simulink model "JOLT"  (R2023a)
settings: Solver=FixedStepAuto  StartTime=0.0  StopTime=2000  RelTol=1e-3
model workspace (MAT data in the model file):
  SampleTime = 0.001
  T_npxls = 4
  T_pupil = 100
  T_whisk = 20
  maxFrames = 60000
  tStop = 1800
  toneDuration = 1.5
undefined symbols (not defined in the file or in its folder): Ended, Single
libraries: speedgoatlib_IO191 x4, slrealtimeiplib x3
settings Model: Creator=electro  LastModifiedBy=electro
settings SolverCC: ConcurrentTasks=on  PositivePriorityOrder=on  AutoInsertRateTranBlk=on
settings DataIOCC: SaveFormat=Array
settings OptimizationCC: BlockReduction=off  OptimizeBlockIOStorage=off  EnhancedBackFolding=on  PassReuseOutputArgsThreshold=0  OptimizeBlockOrder=speed  DifferentSizesBufferReuse=on
settings DebuggingCC: TasksWithSamePriorityMsg=none  ParameterTunabilityLossMsg=error  SFUnexpectedBacktrackingDiag=warning  SFNoUnconditionalDefaultTransitionDiag=warning  UnderSpecifiedDimensionMsg=warning
settings HardwareCC: ProdBitPerLong=64  ProdLongLongMode=on  ProdHWDeviceType=Intel->x86-64 (Linux 64)
settings SFSimCC: SimUserIncludeDirs="\"/usr/local/MATLAB/R2023a/toolbox/slrealtime/target/kernel/dist/include/verify\""
settings RTWCC: Description=Simulink Real-Time  SystemTargetFile=slrealtime.tlc  TemplateMakefile=slrealtime_default_tmf  GenerateReport=on  RTWVerbose=off  CustomInclude=/usr/local/MATLAB/R2023a/toolbox/slrealtime/target/kernel/dist/include,  Toolchain=Simulink Real-Time Toolchain  BuildConfiguration=Faster Runs  CodeExecutionProfiling=on  TargetLang=C++
settings CodeAppCC: ForceParamTrailComments=on  OperatorAnnotations=on  EnableCustomComments=on

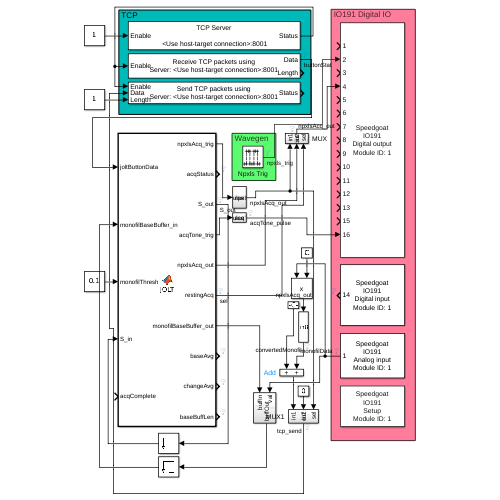
[thumbnail: Simulink's stored preview of the top-level diagram]
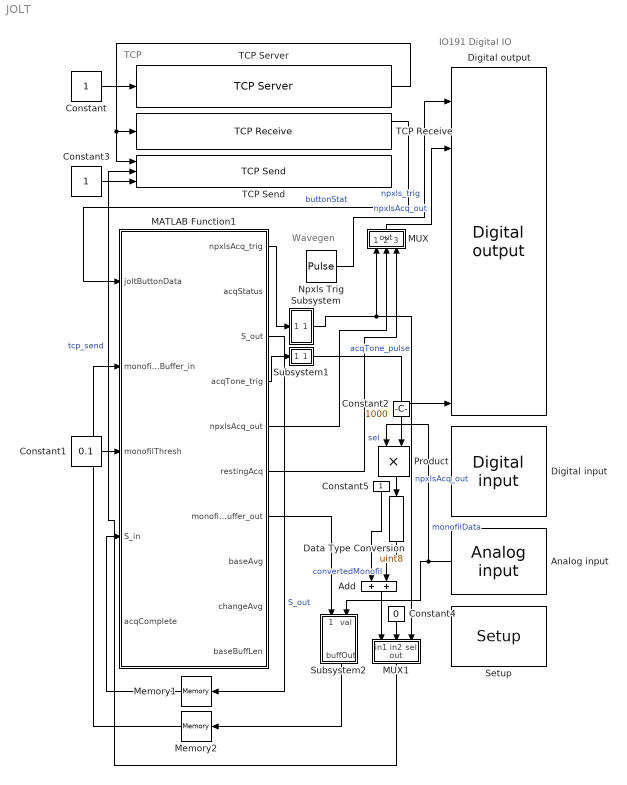
== system JOLT ==
  note: Wavegen
  note: TCP
  note: IO191 Digital IO
  Add : Sum
  "Analog input " : speedgoatlib_IO191/Analog input   parModuleId=1  parSampleTime=SampleTime  parPciSlot=-1  parAdcChannels=1  parAdcMode=2  parAdcRanges=4  parAdcRate=100000  parAdcInitValues=[0 0]  parAdcResets=[1 1]
      settings: SourceProductName=Simulink Real-Time: Speedgoat I/O Blockset
  Constant : Constant
  Constant1 : Constant  Value=0.1
  Constant2 : Constant  Value=1000
  Constant3 : Constant
  Constant4 : Constant  Value=0
  Constant5 : Constant
  Data Type Conversion : DataTypeConversion  OutMin=1  OutMax=255  OutDataTypeStr=uint8  RndMeth=Ceiling  SaturateOnIntegerOverflow=off
  "Digital input " : speedgoatlib_IO191/Digital input   parModuleId=1  parSampleTime=SampleTime  parPciSlot=-1  parDiChannels=14
      settings: SourceProductName=Simulink Real-Time: Speedgoat I/O Blockset
  "Digital output " : speedgoatlib_IO191/Digital output   parModuleId=1  parSampleTime=SampleTime  parPciSlot=-1  parDoChannels=[1 2 3 4 5 6 7 8 9 10 11 12 13 15 16]  parDoInitValues=[1 0 0 0 0 0 0 0 0 0 0 0 0 0 0]  parDoResets=[1 1 1 1 1 1 1 1 1 1 1 1 1 1 1]
      settings: SourceProductName=Simulink Real-Time: Speedgoat I/O Blockset
  MATLAB Function1 : MATLAB Function  TreatAsAtomicUnit=on
  MUX : Subsystem
  MUX1 : Subsystem
  Memory1 : Memory  InheritSampleTime=on
  Memory2 : Memory  InheritSampleTime=on
  Npxls Trig : DiscretePulseGenerator  Amplitude=2.5  Period=T_npxls  PulseWidth=T_npxls/2  SampleTime=SampleTime
  Product : Product
  "Setup " : speedgoatlib_IO191/Setup   parModuleId=1  parPciSlot=-1  parTriggerSignal=TTL  parAdcChannels=1  parAdcRanges=4  parAdcChannel1=on  parAdcChannel2=off  parAdcChannel3=off  parAdcChannel4=off  parAdcChannel5=off  parAdcChannel6=off  parAdcChannel7=off  parAdcChannel8=off  parAdcMode=Single-Ended  parAdcRate=100000  parAdcRange11=+-5.12 V  parAdcRange21=+-24.576 V  parAdcRange12=+-10.24 V  parAdcRange22=+-24.576 V  parAdcRange13=+-10.24 V  parAdcRange23=+-24.576 V  parAdcRange14=+-10.24 V  parAdcRange24=+-24.576 V  parAdcRange15=+-10.24 V  parAdcRange25=+-24.576 V  parAdcRange16=+-10.24 V  parAdcRange26=+-24.576 V  parAdcRange17=+-10.24 V  parAdcRange27=+-24.576 V  parAdcRange18=+-10.24 V  parAdcRange28=+-24.576 V  parDacChannels=[1 2]  parDacChannel1=on  parDacChannel2=on  parDacChannel3=off  parDacChannel4=off  parDacMode=Single-Ended  parDacRanges=[4 4]  parDacInitValues=[0 0]  parDacResets=[1 1]  parDacRange1=+-10 V  parDacInitValue1=0  parDacReset1=on  parDacRange2=+-10 V  parDacInitValue2=0  parDacReset2=on  parDacRange3=+-10 V  parDacInitValue3=0  parDacReset3=on  parDacRange4=+-10 V  parDacInitValue4=0  parDacReset4=on  parDiChannels=14  parDoChannels=[1 2 3 4 5 6 7 8 9 10 11 12 13 15 16]  parDioFirstControl=[1 2 3 4 5 6 8 9]  parDioSecondControl=0  parDioChannel1=Out  parExtra1=I  parExtra2=I  parExtra3=I  parDioChannel2=Out  parDioChannel3=Out  parDioChannel4=Out  parDioChannel5=Out  parDioChannel6=Out  parDioChannel7=In  parDioChannel8=Out  parDioChannel9=Out  parDoInitValues=[0 0 0 0]  parDoResets=[1 1 1 1]  parDoInitValue1=1  parDoReset1=on  parDoInitValue2=0  parDoReset2=on  parDoInitValue3=0  parDoReset3=on  parDoInitValue4=0  parDoReset4=on  parDoInitValue5=0  parDoReset5=on  parDoInitValue6=0  parDoReset6=on  parDoInitValue7=0  parDoReset7=on  parDoInitValue8=0  parDoReset8=on  parDoInitValue9=0  parDoReset9=on  parDoInitValue10=0  parDoReset10=on  parDoInitValue11=0  parDoReset11=on  parDoInitValue12=0  parDoReset12=on  parDoInitValue13=0  parDoReset13=on  parDoInitValue14=0  parDoReset14=on  parDoInitValue15=0  parDoReset15=on  parDoInitValue16=0  parDoReset16=on
      settings: SourceProductName=Simulink Real-Time: Speedgoat I/O Blockset
  Subsystem : Subsystem
  Subsystem1 : Subsystem
  Subsystem2 : Subsystem
  TCP Receive : slrealtimeiplib/TCP Receive  socketAddPortVal=Server: <Use host-target connection>:8001  rcvWidth=1  sampleTime=SampleTime
  TCP Send : slrealtimeiplib/TCP Send  socketAddPortVal=Server: <Use host-target connection>:8001  sampleTime=SampleTime
  TCP Server : slrealtimeiplib/TCP Server  Priority=-1  useHostTargetConn=on  serverAddress=10.10.10.15  serverPort=8001
  wires:
  TCP Receive/1 -> MATLAB Function1/1(joltButtonData)  "buttonStat"
  TCP Server/1 -> TCP Send/1, TCP Receive/1
  Constant/1 -> TCP Server/1
  Npxls Trig/1 -> "Digital output "/2  "npxls_trig"
  "Analog input "/1 -> Subsystem2/2(val), Product/1  "monofilData"
  MATLAB Function1/3(S_out) -> Memory1/1  "S_out"
  Memory1/1 -> MATLAB Function1/4(S_in)
  MATLAB Function1/4(acqTone_trig) -> Subsystem1/1(acqTone_trig)
  Subsystem1/1(sigPulse) -> "Digital output "/15  "acqTone_pulse"
  Constant1/1 -> MATLAB Function1/3(monofilThresh)
  MUX/1(out) -> "Digital output "/4  "npxlsAcq_out"
  Subsystem/1(sigPulse) -> MUX1/3(sel), MUX/1(in1)  "npxlsAcq_out"
  MATLAB Function1/5(npxlsAcq_out) -> MUX/2(in2)
  MATLAB Function1/6(restingAcq) -> MUX/3(sel)  "sel"
  MATLAB Function1/1(npxlsAcq_trig) -> Subsystem/1(npxlsAcq_trig)
  MATLAB Function1/7(monofilBaseBuffer_out) -> Subsystem2/1(buffIn)
  Subsystem2/1(buffOut) -> Memory2/1
  Memory2/1 -> MATLAB Function1/2(monofilBaseBuffer_in)
  Constant2/1 -> Product/2
  Constant3/1 -> TCP Send/3
  Constant4/1 -> MUX1/2(in2)
  MUX1/1(out) -> TCP Send/2  "tcp_send"
  Constant5/1 -> Add/1
  Product/1 -> Data Type Conversion/1
  Add/1 -> MUX1/1(in1)
  Data Type Conversion/1 -> Add/2  "convertedMonofil"

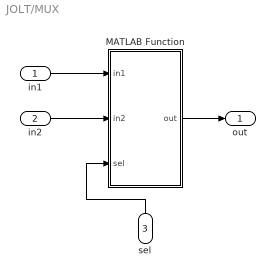
== system JOLT/MUX ==
  in1 : Inport
  in2 : Inport  Port=2
  sel : Inport  Port=3
  MATLAB Function : MATLAB Function  TreatAsAtomicUnit=on
  out : Outport
  wires:
  in1/1 -> MATLAB Function/1(in1)
  in2/1 -> MATLAB Function/2(in2)
  sel/1 -> MATLAB Function/3(sel)
  MATLAB Function/1(out) -> out/1

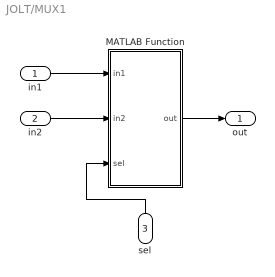
== system JOLT/MUX1 ==
  in1 : Inport
  in2 : Inport  Port=2
  sel : Inport  Port=3
  MATLAB Function : MATLAB Function  TreatAsAtomicUnit=on
  out : Outport
  wires:
  in1/1 -> MATLAB Function/1(in1)
  in2/1 -> MATLAB Function/2(in2)
  sel/1 -> MATLAB Function/3(sel)
  MATLAB Function/1(out) -> out/1

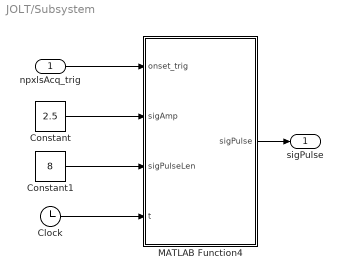
== system JOLT/Subsystem ==
  npxlsAcq_trig : Inport
  Clock : Clock
  Constant : Constant  Value=2.5
  Constant1 : Constant  Value=8
  MATLAB Function4 : MATLAB Function  TreatAsAtomicUnit=on
  sigPulse : Outport
  wires:
  npxlsAcq_trig/1 -> MATLAB Function4/1(onset_trig)
  MATLAB Function4/1(sigPulse) -> sigPulse/1
  Constant/1 -> MATLAB Function4/2(sigAmp)
  Constant1/1 -> MATLAB Function4/3(sigPulseLen)
  Clock/1 -> MATLAB Function4/4(t)

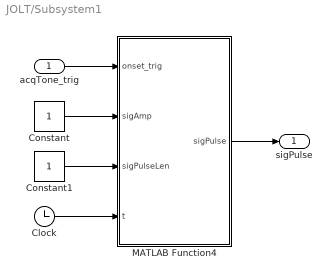
== system JOLT/Subsystem1 ==
  acqTone_trig : Inport
  Clock : Clock
  Constant : Constant
  Constant1 : Constant
  MATLAB Function4 : MATLAB Function  TreatAsAtomicUnit=on
  sigPulse : Outport
  wires:
  acqTone_trig/1 -> MATLAB Function4/1(onset_trig)
  MATLAB Function4/1(sigPulse) -> sigPulse/1
  Clock/1 -> MATLAB Function4/4(t)
  Constant/1 -> MATLAB Function4/2(sigAmp)
  Constant1/1 -> MATLAB Function4/3(sigPulseLen)

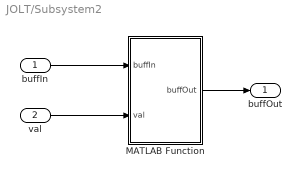
== system JOLT/Subsystem2 ==
  buffIn : Inport
  val : Inport  Port=2
  MATLAB Function : MATLAB Function  TreatAsAtomicUnit=on
  buffOut : Outport  PortDimensions=[1,10000]
  wires:
  buffIn/1 -> MATLAB Function/1(buffIn)
  val/1 -> MATLAB Function/2(val)
  MATLAB Function/1(buffOut) -> buffOut/1

== matlab function JOLT/MUX/MATLAB Function ==
  data: in1 input; out output; in2 input; sel input
function out = MUX(in1, in2, sel)
    switch sel
        case 1
            out = in1;
        case 2
            out = in2;    
        otherwise
            out = 0;
    end
end

== matlab function JOLT/MATLAB Function1 ==
  data: npxlsAcq_trig output; acqStatus output; S_out output; joltButtonData input; monofilBaseBuffer_in input; monofilThresh input; acqTone_trig output; S_in input; acqComplete input; npxlsAcq_out output; restingAcq output; monofilBaseBuffer_out output; baseAvg output; changeAvg output; baseBuffLen output
function [npxlsAcq_trig, acqStatus, S_out, acqTone_trig, npxlsAcq_out, restingAcq, monofilBaseBuffer_out, baseAvg, changeAvg, baseBuffLen] = JOLT(joltButtonData, monofilBaseBuffer_in, monofilThresh, S_in, acqComplete)
    
    monofilBaseBufferLEN = 10000;
    monofilChangeBufferLEN = 50;   
    
    
    %% JOLT STATE MACHINE; {S0 - rest, S1 - monofilTrack, S2 - acquire}
    switch S_in
        case 0 % Resting state (respond to buttons)            
            switch uint8(joltButtonData)
                case 1 % trial start
                    npxlsAcq_out=0;
                    acqStatus=1;                    
                    S_out = 1;
                    restingAcq=0;
                case 2 % trial save
                    npxlsAcq_out=0;
                    acqStatus=2;
                    S_out = S_in;
                    restingAcq=0;
                case 3 % trial discard
                    npxlsAcq_out=0;
                    acqStatus=3;
                    S_out = S_in;
                    restingAcq=0;
                case 4 % resting acquisition
                    acqStatus=4;
                    restingAcq=2;
                    npxlsAcq_out=2.5;
                    S_out=0;                    
                otherwise
                    % npxlsAcq_out = npxlsAcq_in;
                    acqStatus=0;
                    S_out = S_in;
                    npxlsAcq_out=0;
                    restingAcq=0;
            end 
            acqTone_trig=0;
            npxlsAcq_trig=0;
            baseAvg=0;
            changeAvg=0;
            baseBuffLen=0;
            monofilBaseBuffer_out=zeros(1,monofilBaseBufferLEN);
        case 1 % track monofilament
            acqStatus=0;
            acqTone_trig=0;
            npxlsAcq_out=0;
            npxlsAcq_trig=0;
            restingAcq=0;
            % while true
            % baseAvg=0;
            % changeAvg=0;
            S_out=1;
            % queue monofil baseline buffer
            % monofilBaseBuffer_out = [monofilBaseBuffer, monofilData];                
            % monofilBaseBuffer_out=zeros(1,monofilBaseBufferLEN);
            if length(monofilBaseBuffer_in) > monofilBaseBufferLEN
                monofilBaseBuffer_out = monofilBaseBuffer_in(2:end);
            else
                monofilBaseBuffer_out = monofilBaseBuffer_in;
            end
            baseBuffLen = length(monofilBaseBuffer_out);
            if baseBuffLen == monofilBaseBufferLEN % if buffer full and ready for avging
                % calc base avg
                baseAvg = mean(nonzeros(monofilBaseBuffer_out((baseBuffLen+1)-monofilBaseBufferLEN:end)));
                % calc change avg
                changeAvg = mean(nonzeros(monofilBaseBuffer_out((baseBuffLen+1)-monofilChangeBufferLEN:end)));
                % poll for acquisition cue
                if changeAvg > (baseAvg*3)
                    S_out=2; % change to 'acquire' state
                    % break;
                end
            end                             
            % end            
        case 2 % Acquisition state (hold acq for T seconds and then rest)
            monofilBaseBuffer_out=monofilBaseBuffer_in;
            baseBuffLen=0;
            baseAvg=0;
            changeAvg=0;
            acqStatus=0;
            restingAcq=0;
            npxlsAcq_out=0;            
            npxlsAcq_trig = 1;
            acqTone_trig = 1; % sound the acquisition            
            S_out = 0; % return to resting           
        otherwise
            monofilBaseBuffer_out=monofilBaseBuffer_in;
            baseBuffLen=0;
            baseAvg=0;
            changeAvg=0;
            S_out = 0;            
            acqStatus = 0;
            acqTone_trig = 0;
            npxlsAcq_out=0;
            npxlsAcq_trig=0;
            restingAcq=1;
    end
end

== matlab function JOLT/Subsystem2/MATLAB Function ==
  data: buffOut output; buffIn input; val input
function buffOut = buffer(buffIn, val)
    buffOut = signalBuffer(2, buffIn, val);
end

== matlab function JOLT/Subsystem/MATLAB Function4 ==
  data: onset_trig input; sigAmp input; sigPulseLen input; sigPulse output; t input
function sigPulse   = holdSig(onset_trig, sigAmp, sigPulseLen, t) 
   sigPulse = holdSignal(onset_trig, sigAmp, sigPulseLen, t);
end

== matlab function JOLT/Subsystem1/MATLAB Function4 ==
  data: onset_trig input; sigAmp input; sigPulseLen input; sigPulse output; t input
function sigPulse  = holdSig(onset_trig, sigAmp, sigPulseLen, t) 
   sigPulse = holdSignal(onset_trig, sigAmp, sigPulseLen, t);
end

== matlab function JOLT/MUX1/MATLAB Function ==
  data: in1 input; out output; in2 input; sel input
function out = MUX(in1, in2, sel)
    switch sel
        case 0
            out = uint8(in1);
        % case 2.5
        %     out = uint8(in2);    
        otherwise
            out = uint8(in2);
    end
end
